simulink model "state1"  (R2015a)
settings: Solver=ode3  StartTime=0.0  StopTime=10.0  RelTol=1e-3
libraries: legoev3lib x4, simulink x1
settings Model: SimulationMode=external  ExtModeTrigDuration=2  Creator=USER  LastModifiedBy=USER
settings OptimizationCC: OptimizeModelRefInitCode=on  LifeSpan=1
settings DebuggingCC: UnderspecifiedInitializationDetection=Classic  MergeDetectMultiDrivingBlocksExec=none
settings HardwareCC: ProdLargestAtomicInteger=Long  ProdLargestAtomicFloat=Float  ProdEndianess=LittleEndian  ProdHWDeviceType=ARM Compatible->ARM 9
settings RTWCC: SystemTargetFile=realtime.tlc  GenerateMakefile=off  TemplateMakefile=realtime.tmf  Description=Run on Target Hardware  RTWVerbose=off
settings ERTTargetCC: CombineOutputUpdateFcns=off  ERTSrcFileBannerTemplate=realtime_code_template.cgt  ERTHdrFileBannerTemplate=realtime_code_template.cgt  ERTDataSrcFileTemplate=realtime_code_template.cgt  ERTDataHdrFileTemplate=realtime_code_template.cgt  ERTCustomFileTemplate=realtime_file_process.tlc

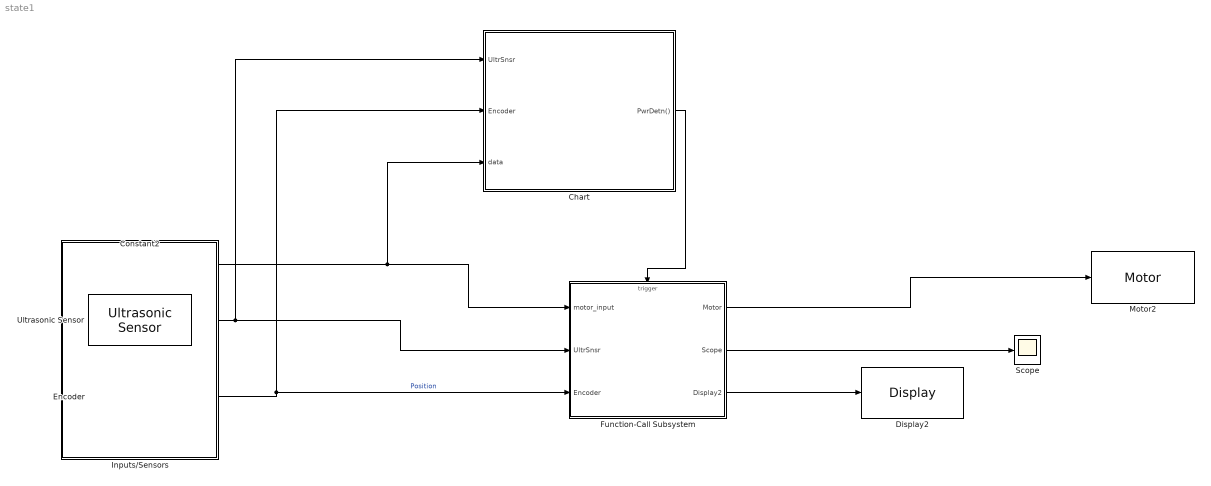
== system state1 ==
  Chart : Stateflow chart  TreatAsAtomicUnit=on
  Constant2 : Constant  Value=20
  Display2 : legoev3lib/Display  slcdStr=Obj_Det  slcdLine=1  slcdFormat=Decimal
  Encoder : legoev3lib/Encoder  portNumber=A  opMode=No reset  sampleTime=0.01
  Function-Call Subsystem : Subsystem  TreatAsAtomicUnit=on
  Inputs/Sensors : Subsystem
  Motor2 : legoev3lib/Motor  sportNumber=A  sstopAction=Brake
  Scope : Scope
      settings: YMin=-90  YMax=80  SaveName=acqData
  Ultrasonic Sensor : legoev3lib/Ultrasonic Sensor  PortNumber=1  sampleTime=0.01
  wires:
  Ultrasonic Sensor/1 -> Chart/1(UltrSnsr), Function-Call Subsystem/2(UltrSnsr)
  Constant2/1 -> Chart/3(data), Function-Call Subsystem/1(motor_input)
  Function-Call Subsystem/3(Display2) -> Display2/1
  Function-Call Subsystem/2(Scope) -> Scope/1
  Function-Call Subsystem/1(Motor) -> Motor2/1
  Encoder/1 -> Chart/2(Encoder), Function-Call Subsystem/3(Encoder)  "Position"
  Chart/1(PwrDetn()) -> Function-Call Subsystem/Trigger

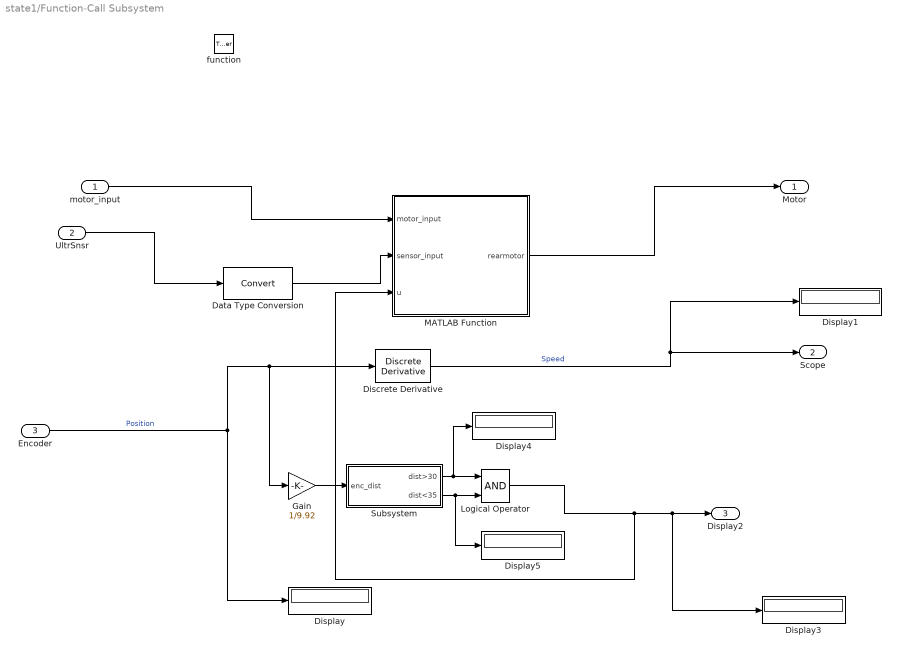
== system state1/Function-Call Subsystem ==
  motor_input : Inport
  UltrSnsr : Inport  Port=2
  Encoder : Inport  Port=3
  function : TriggerPort  TriggerType=function-call
  Data Type Conversion : DataTypeConversion
  Discrete Derivative : simulink/Discrete/Discrete Derivative  gainval=1.0  ICPrevScaledInput=800  InputProcessing=Inherited  OutMin=[]  OutMax=[]  OutDataTypeStr=double  OutputDataTypeScalingMode=double  OutDataType=fixdt(1, 16)  OutScaling=2^-10  DoSatur=off
  Display{,1,3..5} (5 alike) : Display
  Gain : Gain  Gain=1/9.92
  Logical Operator : Logic  AllPortsSameDT=off  OutDataTypeStr=boolean
  MATLAB Function : MATLAB Function  TreatAsAtomicUnit=on
  Subsystem : Subsystem
  Motor : Outport
  Scope : Outport  Port=2
  Display2 : Outport  Port=3
  wires:
  Data Type Conversion/1 -> MATLAB Function/2(sensor_input)
  MATLAB Function/1(rearmotor) -> Motor/1
  Encoder/1 -> Gain/1, Discrete Derivative/1, Display/1  "Position"
  UltrSnsr/1 -> Data Type Conversion/1
  Discrete Derivative/1 -> Display1/1, Scope/1  "Speed"
  Gain/1 -> Subsystem/1(enc_dist)
  Subsystem/1(dist>30) -> Display4/1, Logical Operator/1
  Subsystem/2(dist<35) -> Display5/1, Logical Operator/2
  Logical Operator/1 -> MATLAB Function/3(u), Display3/1, Display2/1
  motor_input/1 -> MATLAB Function/1(motor_input)

== system state1/Inputs//Sensors ==

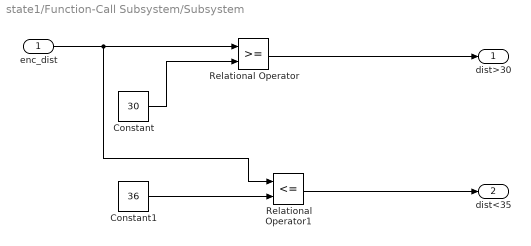
== system state1/Function-Call Subsystem/Subsystem ==
  enc_dist : Inport
  Constant : Constant  Value=30
  Constant1 : Constant  Value=36
  Relational Operator : RelationalOperator  OutDataTypeStr=boolean
  Relational Operator1 : RelationalOperator  Operator=<=  OutDataTypeStr=boolean
  dist>30 : Outport
  dist<35 : Outport  Port=2
  wires:
  enc_dist/1 -> Relational Operator1/1, Relational Operator/1
  Constant/1 -> Relational Operator/2
  Constant1/1 -> Relational Operator1/2
  Relational Operator/1 -> dist>30/1
  Relational Operator1/1 -> dist<35/1

== matlab function state1/Function-Call Subsystem/MATLAB Function ==
  data: motor_input input; sensor_input input; rearmotor output; u input
function rearmotor = fcn(motor_input,sensor_input,u)
%#codegen
if(sensor_input>4)&&(sensor_input<=20)&& (u==1)
    rearmotor=motor_input;
%elseif(sensor_input>20)&&(sensor_input<=35)
 %   rearmotor=motor_input;
else
    rearmotor=0;
end
end

== stateflow chart state1/Chart ==
  state ParkSpotDectd
    du: send(PwrDetn);
  (default) -> ParkSpotDectd
  data: UltrSnsr input; Encoder input; data input
  events: PwrDetn output FUNCTION_CALL_EVENT; wait local RISING_EDGE_EVENT
